simulink model "Hierarchical_Scheduler_2"  (Simulink 7.3)
settings: Solver=ode45  StartTime=0.0  StopTime=35000  RelTol=1e-3
model workspace: external: M-Code (data not in the file)
undefined symbols (not defined in the file or in its folder): D1, D2, D3, DiscIntNeverNeededParam, Sub, T1, T2, T3
libraries: simulink x3
settings Model: Creator=nmd01  LastModifiedBy=nmd01

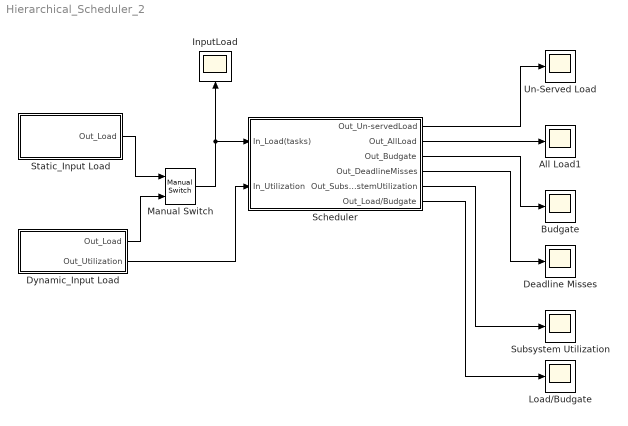
== system Hierarchical_Scheduler_2 ==
  All Load1 : Scope
      settings: SaveName=Utilization1  DataFormat=Array
  Budgate : Scope
      settings: SaveName=Utilization2  DataFormat=Array
  Deadline Misses : Scope
      settings: SaveName=Utilization11  DataFormat=Array
  Dynamic_Input Load : Subsystem
  InputLoad : Scope
      settings: SaveName=Utilization3  DataFormat=Array
  Load/Budgate : Scope
      settings: SaveName=Utilization13  DataFormat=Array
  Manual Switch : simulink/Signal Routing/Manual Switch  SystemSampleTime=-1  sw=1  action=0  varsize=off
  Scheduler : Subsystem
  Static_Input Load : Subsystem
  Subsystem Utilization : Scope
      settings: SaveName=Utilization12  DataFormat=Array
  Un-Served Load : Scope
      settings: SaveName=h  DataFormat=Array
  wires:
  Scheduler/1(Out_Un-servedLoad) -> Un-Served Load/1
  Scheduler/3(Out_Budgate) -> Budgate/1
  Static_Input Load/1(Out_Load) -> Manual Switch/1
  Dynamic_Input Load/1(Out_Load) -> Manual Switch/2
  Manual Switch/1 -> Scheduler/1(In_Load(tasks)), InputLoad/1
  Dynamic_Input Load/2(Out_Utilization) -> Scheduler/2(In_Utilization)
  Scheduler/4(Out_DeadlineMisses) -> Deadline Misses/1
  Scheduler/5(Out_SubsystemUtilization) -> Subsystem Utilization/1
  Scheduler/2(Out_AllLoad) -> All Load1/1
  Scheduler/6(Out_Load/Budgate) -> Load/Budgate/1

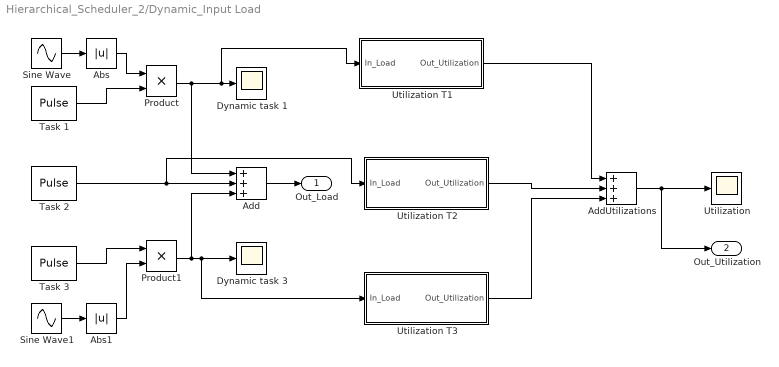
== system Hierarchical_Scheduler_2/Dynamic_Input Load ==
  Abs : Abs  OutDataType=fixdt(1, 16)  OutScaling=2^0
  Abs1 : Abs  OutDataType=fixdt(1, 16)  OutScaling=2^0
  Add : Sum  Inputs=+++  OutDataType=fixdt(1, 16)  OutScaling=2^-10
  AddUtilizations : Sum  Inputs=+++  OutDataType=fixdt(1, 16)  OutScaling=2^-10
  Dynamic task 1 : Scope
      settings: SaveName=Utilization6  DataFormat=Array
  Dynamic task 3 : Scope
      settings: SaveName=Utilization7  DataFormat=Array
  Product : Product  OutDataType=fixdt(1, 16)  OutScaling=2^0  SampleTime=1  RndMeth=Zero
  Product1 : Product  OutDataType=fixdt(1, 16)  OutScaling=2^0  SampleTime=1  RndMeth=Zero
  Sine Wave : Sin  Amplitude=1  Bias=0  Frequency=1  Phase=0  Samples=10  SampleTime=0  Offset=0
  Sine Wave1 : Sin  Amplitude=1  Bias=0  Frequency=3  Phase=0  Samples=10  SampleTime=0  Offset=0
  Task 1 : DiscretePulseGenerator  PulseType=Time based  Amplitude=5  Period=T1  PulseWidth=1  PhaseDelay=D1  SampleTime=1
  Task 2 : DiscretePulseGenerator  PulseType=Time based  Amplitude=2  Period=T2  PulseWidth=1  PhaseDelay=D2  SampleTime=1
  Task 3 : DiscretePulseGenerator  PulseType=Time based  Amplitude=1  Period=T3  PulseWidth=1  PhaseDelay=D3  SampleTime=1
  Utilization : Scope
      settings: SaveName=Utilization8  DataFormat=Array
  Utilization T1 : Subsystem
  Utilization T2 : Subsystem
  Utilization T3 : Subsystem
  Out_Load : Outport  OutDataType=fixdt(1, 16)  OutScaling=2^0
  Out_Utilization : Outport  Port=2  OutDataType=fixdt(1, 16)  OutScaling=2^0
  wires:
  Add/1 -> Out_Load/1
  Task 2/1 -> Add/2, Utilization T2/1(In_Load)
  Sine Wave/1 -> Abs/1
  Abs/1 -> Product/1
  Task 1/1 -> Product/2
  Product/1 -> Add/1, Dynamic task 1/1, Utilization T1/1(In_Load)
  Sine Wave1/1 -> Abs1/1
  Task 3/1 -> Product1/1
  Abs1/1 -> Product1/2
  Product1/1 -> Add/3, Dynamic task 3/1, Utilization T3/1(In_Load)
  Utilization T1/1(Out_Utilization) -> AddUtilizations/1
  Utilization T2/1(Out_Utilization) -> AddUtilizations/2
  Utilization T3/1(Out_Utilization) -> AddUtilizations/3
  AddUtilizations/1 -> Utilization/1, Out_Utilization/1

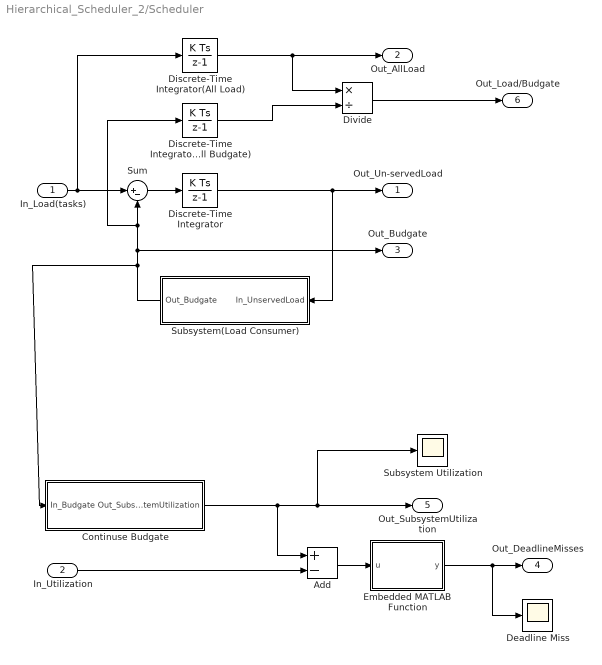
== system Hierarchical_Scheduler_2/Scheduler ==
  In_Load(tasks) : Inport  OutDataType=fixdt(1, 16)  OutScaling=2^0
  In_Utilization : Inport  Port=2  OutDataType=fixdt(1, 16)  OutScaling=2^0
  Add : Sum  Inputs=+-  OutDataType=fixdt(1, 16)  OutScaling=2^-10
  Continuse Budgate : Subsystem
  Deadline Miss : Scope
      settings: SaveName=Utilization10  DataFormat=Array
  Discrete-Time Integrator : DiscreteIntegrator  OutDataType=fixdt(1, 16)  OutScaling=2^0  LimitOutput=on  LowerSaturationLimit=0  ICPrevOutput=DiscIntNeverNeededParam  ICPrevScaledInput=DiscIntNeverNeededParam
  Discrete-Time Integrator(All Budgate) : DiscreteIntegrator  OutDataType=fixdt(1, 16)  OutScaling=2^0  LowerSaturationLimit=0  ICPrevOutput=DiscIntNeverNeededParam  ICPrevScaledInput=DiscIntNeverNeededParam
  Discrete-Time Integrator(All Load) : DiscreteIntegrator  OutDataType=fixdt(1, 16)  OutScaling=2^0  LowerSaturationLimit=0  ICPrevOutput=DiscIntNeverNeededParam  ICPrevScaledInput=DiscIntNeverNeededParam
  Divide : Product  Inputs=*/  OutDataType=fixdt(1, 16)  OutScaling=2^-10
  Embedded MATLAB Function : Stateflow chart
  Subsystem Utilization : Scope
      settings: SaveName=Utilization9  DataFormat=Array
  Subsystem(Load Consumer) : Subsystem
  Sum : Sum  Inputs=|+-  OutDataType=fixdt(1, 16)  OutScaling=2^0  SampleTime=1
  Out_Un-servedLoad : Outport  OutDataType=fixdt(1, 16)  OutScaling=2^0
  Out_AllLoad : Outport  Port=2  OutDataType=fixdt(1, 16)  OutScaling=2^0
  Out_Budgate : Outport  Port=3  OutDataType=fixdt(1, 16)  OutScaling=2^0
  Out_DeadlineMisses : Outport  Port=4  OutDataType=fixdt(1, 16)  OutScaling=2^0
  Out_SubsystemUtilization : Outport  Port=5  OutDataType=fixdt(1, 16)  OutScaling=2^0
  Out_Load/Budgate : Outport  Port=6  OutDataType=fixdt(1, 16)  OutScaling=2^0
  wires:
  In_Load(tasks)/1 -> Sum/1, Discrete-Time Integrator(All Load)/1
  Sum/1 -> Discrete-Time Integrator/1
  Discrete-Time Integrator/1 -> Out_Un-servedLoad/1, Subsystem(Load Consumer)/1(In_UnservedLoad)
  Subsystem(Load Consumer)/1(Out_Budgate) -> Out_Budgate/1, Sum/2, Discrete-Time Integrator(All Budgate)/1, Continuse Budgate/1(In_Budgate)
  Continuse Budgate/1(Out_SubsystemUtilization) -> Add/1, Subsystem Utilization/1, Out_SubsystemUtilization/1
  In_Utilization/1 -> Add/2
  Discrete-Time Integrator(All Load)/1 -> Out_AllLoad/1, Divide/1
  Divide/1 -> Out_Load/Budgate/1
  Discrete-Time Integrator(All Budgate)/1 -> Divide/2
  Add/1 -> Embedded MATLAB Function/1(u)
  Embedded MATLAB Function/1(y) -> Out_DeadlineMisses/1, Deadline Miss/1

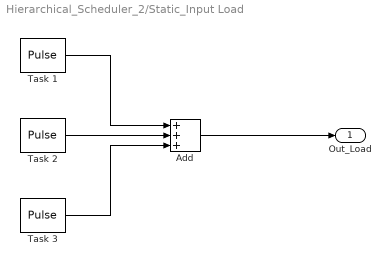
== system Hierarchical_Scheduler_2/Static_Input Load ==
  Add : Sum  Inputs=+++  OutDataType=fixdt(1, 16)  OutScaling=2^-10
  Task 1 : DiscretePulseGenerator  PulseType=Time based  Amplitude=3  Period=T1  PulseWidth=1  PhaseDelay=D1  SampleTime=1
  Task 2 : DiscretePulseGenerator  PulseType=Time based  Amplitude=2  Period=T2  PulseWidth=1  PhaseDelay=D2  SampleTime=1
  Task 3 : DiscretePulseGenerator  PulseType=Time based  Amplitude=1  Period=T3  PulseWidth=D3  PhaseDelay=0  SampleTime=1
  Out_Load : Outport  OutDataType=fixdt(1, 16)  OutScaling=2^0
  wires:
  Add/1 -> Out_Load/1
  Task 1/1 -> Add/1
  Task 2/1 -> Add/2
  Task 3/1 -> Add/3

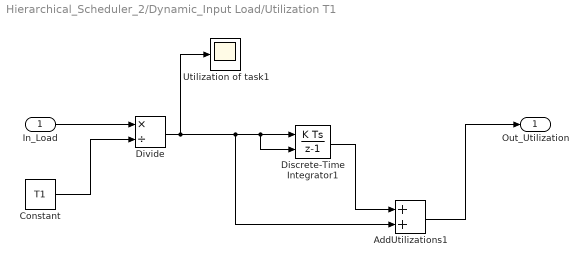
== system Hierarchical_Scheduler_2/Dynamic_Input Load/Utilization T1 ==
  In_Load : Inport  OutDataType=fixdt(1, 16)  OutScaling=2^0
  AddUtilizations1 : Sum  OutDataType=fixdt(1, 16)  OutScaling=2^-10
  Constant : Constant  Value=T1  OutDataType=fixdt(1, 16)  OutScaling=2^0
  Discrete-Time Integrator1 : DiscreteIntegrator  ExternalReset=rising  OutDataType=fixdt(1, 16)  OutScaling=2^0  ICPrevOutput=DiscIntNeverNeededParam  ICPrevScaledInput=DiscIntNeverNeededParam
  Divide : Product  Inputs=*/  OutDataType=fixdt(1, 16)  OutScaling=2^-10
  Utilization of task1 : Scope
      settings: SaveName=Utilization  DataFormat=Array
  Out_Utilization : Outport  OutDataType=fixdt(1, 16)  OutScaling=2^0
  wires:
  In_Load/1 -> Divide/1
  Constant/1 -> Divide/2
  Divide/1 -> Discrete-Time Integrator1/1, Discrete-Time Integrator1/2, AddUtilizations1/2, Utilization of task1/1
  Discrete-Time Integrator1/1 -> AddUtilizations1/1
  AddUtilizations1/1 -> Out_Utilization/1

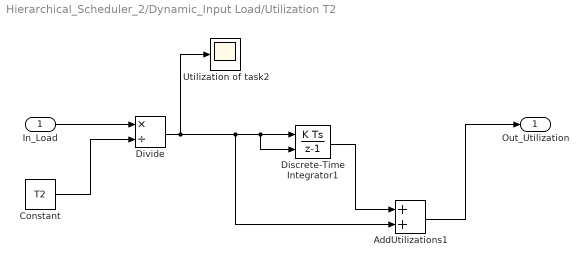
== system Hierarchical_Scheduler_2/Dynamic_Input Load/Utilization T2 ==
  In_Load : Inport  OutDataType=fixdt(1, 16)  OutScaling=2^0
  AddUtilizations1 : Sum  OutDataType=fixdt(1, 16)  OutScaling=2^-10
  Constant : Constant  Value=T2  OutDataType=fixdt(1, 16)  OutScaling=2^0
  Discrete-Time Integrator1 : DiscreteIntegrator  ExternalReset=rising  OutDataType=fixdt(1, 16)  OutScaling=2^0  ICPrevOutput=DiscIntNeverNeededParam  ICPrevScaledInput=DiscIntNeverNeededParam
  Divide : Product  Inputs=*/  OutDataType=fixdt(1, 16)  OutScaling=2^-10
  Utilization of task2 : Scope
      settings: SaveName=Utilization  DataFormat=Array
  Out_Utilization : Outport  OutDataType=fixdt(1, 16)  OutScaling=2^0
  wires:
  AddUtilizations1/1 -> Out_Utilization/1
  Discrete-Time Integrator1/1 -> AddUtilizations1/1
  Divide/1 -> Utilization of task2/1, AddUtilizations1/2, Discrete-Time Integrator1/2, Discrete-Time Integrator1/1
  Constant/1 -> Divide/2
  In_Load/1 -> Divide/1

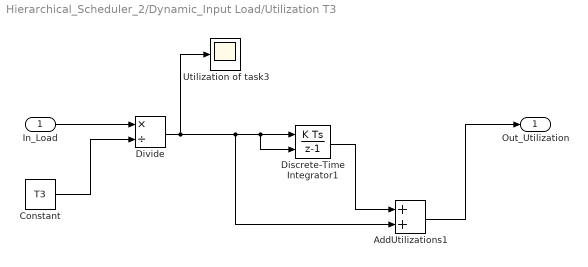
== system Hierarchical_Scheduler_2/Dynamic_Input Load/Utilization T3 ==
  In_Load : Inport  OutDataType=fixdt(1, 16)  OutScaling=2^0
  AddUtilizations1 : Sum  OutDataType=fixdt(1, 16)  OutScaling=2^-10
  Constant : Constant  Value=T3  OutDataType=fixdt(1, 16)  OutScaling=2^0
  Discrete-Time Integrator1 : DiscreteIntegrator  ExternalReset=rising  OutDataType=fixdt(1, 16)  OutScaling=2^0  ICPrevOutput=DiscIntNeverNeededParam  ICPrevScaledInput=DiscIntNeverNeededParam
  Divide : Product  Inputs=*/  OutDataType=fixdt(1, 16)  OutScaling=2^-10
  Utilization of task3 : Scope
      settings: SaveName=Utilization  DataFormat=Array
  Out_Utilization : Outport  OutDataType=fixdt(1, 16)  OutScaling=2^0
  wires:
  In_Load/1 -> Divide/1
  Constant/1 -> Divide/2
  Divide/1 -> Discrete-Time Integrator1/1, Discrete-Time Integrator1/2, AddUtilizations1/2, Utilization of task3/1
  Discrete-Time Integrator1/1 -> AddUtilizations1/1
  AddUtilizations1/1 -> Out_Utilization/1

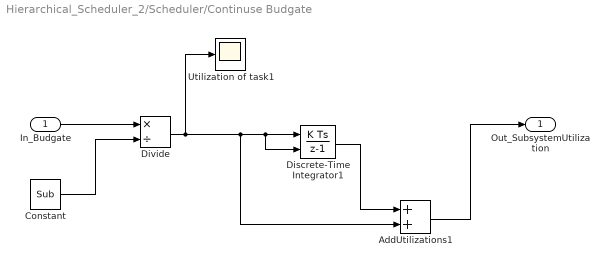
== system Hierarchical_Scheduler_2/Scheduler/Continuse Budgate ==
  In_Budgate : Inport  OutDataType=fixdt(1, 16)  OutScaling=2^0
  AddUtilizations1 : Sum  OutDataType=fixdt(1, 16)  OutScaling=2^-10
  Constant : Constant  Value=Sub  OutDataType=fixdt(1, 16)  OutScaling=2^0
  Discrete-Time Integrator1 : DiscreteIntegrator  ExternalReset=rising  OutDataType=fixdt(1, 16)  OutScaling=2^0  ICPrevOutput=DiscIntNeverNeededParam  ICPrevScaledInput=DiscIntNeverNeededParam
  Divide : Product  Inputs=*/  OutDataType=fixdt(1, 16)  OutScaling=2^-10
  Utilization of task1 : Scope
      settings: SaveName=Utilization  DataFormat=Array
  Out_SubsystemUtilization : Outport  OutDataType=fixdt(1, 16)  OutScaling=2^0
  wires:
  In_Budgate/1 -> Divide/1
  Discrete-Time Integrator1/1 -> AddUtilizations1/1
  AddUtilizations1/1 -> Out_SubsystemUtilization/1
  Divide/1 -> Discrete-Time Integrator1/1, Discrete-Time Integrator1/2, AddUtilizations1/2, Utilization of task1/1
  Constant/1 -> Divide/2

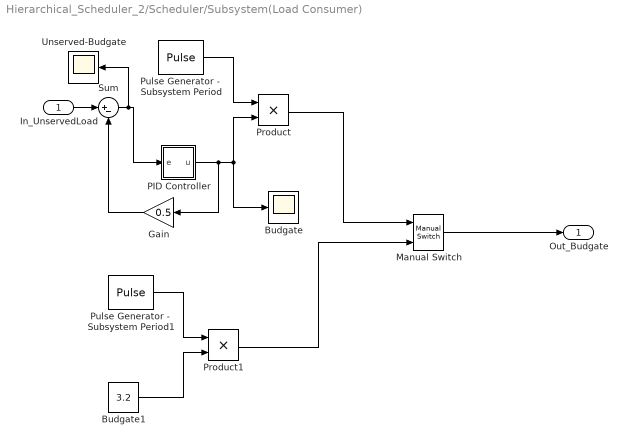
== system Hierarchical_Scheduler_2/Scheduler/Subsystem(Load Consumer) ==
  In_UnservedLoad : Inport  OutDataType=fixdt(1, 16)  OutScaling=2^0
  Budgate : Scope
      settings: SaveName=Utilization4  DataFormat=Array
  Budgate1 : Constant  Value=3.2  OutDataType=fixdt(1, 16)  OutScaling=2^0
  Gain : Gain  Gain=0.5  ParameterDataType=fixdt(1, 16)  ParameterScaling=2^0  OutDataType=fixdt(1, 16)  OutScaling=2^0
  Manual Switch : simulink/Signal Routing/Manual Switch  SystemSampleTime=-1  sw=1  action=0  varsize=off
  PID Controller : Subsystem  AncestorBlock=simulink_extras/Additional Linear/PID Controller  mask(PID Controller){P=.01, I=.001, D=0}
      mask prompts: P "Proportional:"; I "Integral:"; D "Derivative:"
      mask help:
      | Enter expressions for proportional, integral, and derivative terms.
      | P+I/s+Ds
      mask Help: This block implements a PID controller where parameters are entered for the Proportional, Integral and Derivative terms. Unmask this block to see how it works. The derivative term is implemented using a true derivative block.
      mask Display: disp('PID')
  Product : Product  OutDataType=fixdt(1, 16)  OutScaling=2^0  SampleTime=1  RndMeth=Zero
  Product1 : Product  OutDataType=fixdt(1, 16)  OutScaling=2^0  SampleTime=1  RndMeth=Zero
  Pulse Generator -  Subsystem Period : DiscretePulseGenerator  PulseType=Time based  Amplitude=1  Period=Sub  PulseWidth=1  PhaseDelay=0  SampleTime=1
  Pulse Generator -  Subsystem Period1 : DiscretePulseGenerator  PulseType=Time based  Amplitude=1  Period=Sub  PulseWidth=1  PhaseDelay=0  SampleTime=1
  Sum : Sum  Inputs=|+-  OutDataType=fixdt(1, 16)  OutScaling=2^0  SampleTime=1
  Unserved-Budgate : Scope
      settings: SaveName=Utilization5  DataFormat=Array
  Out_Budgate : Outport  OutDataType=fixdt(1, 16)  OutScaling=2^0
  wires:
  Pulse Generator -  Subsystem Period/1 -> Product/1
  PID Controller/1(u) -> Product/2, Budgate/1, Gain/1
  In_UnservedLoad/1 -> Sum/1
  Sum/1 -> PID Controller/1(e), Unserved-Budgate/1
  Pulse Generator -  Subsystem Period1/1 -> Product1/1
  Budgate1/1 -> Product1/2
  Product/1 -> Manual Switch/1
  Product1/1 -> Manual Switch/2
  Manual Switch/1 -> Out_Budgate/1
  Gain/1 -> Sum/2

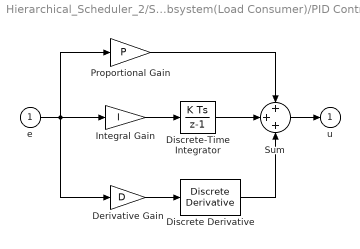
== system Hierarchical_Scheduler_2/Scheduler/Subsystem(Load Consumer)/PID Controller ==
  e : Inport  OutDataType=sfix(16)  OutScaling=2^0
  Derivative Gain : Gain  Gain=D  ParameterDataType=sfix(16)  ParameterScaling=2^0  OutDataType=sfix(16)  OutScaling=2^0  SampleTime=Sub  SaturateOnIntegerOverflow=on  OutDataTypeStr=Inherit: Same as input  ParamDataTypeStr=Inherit: Same as input
  Discrete Derivative : simulink/Discrete/Discrete Derivative  SystemSampleTime=-1  gainval=1.0  ICPrevScaledInput=0.0  OutMin=[]  OutMax=[]  OutDataType=fixdt(1, 16)  OutScaling=2^-10  DoSatur=off
  Discrete-Time Integrator : DiscreteIntegrator  InitialCondition=1  SampleTime=Sub  OutDataType=fixdt(1, 16)  OutScaling=2^0  ICPrevOutput=DiscIntNeverNeededParam  ICPrevScaledInput=DiscIntNeverNeededParam
  Integral Gain : Gain  Gain=I  ParameterDataType=sfix(16)  ParameterScaling=2^0  OutDataType=sfix(16)  OutScaling=2^0  SampleTime=Sub  SaturateOnIntegerOverflow=on  OutDataTypeStr=Inherit: Same as input  ParamDataTypeStr=Inherit: Same as input
  Proportional Gain : Gain  Gain=P  ParameterDataType=sfix(16)  ParameterScaling=2^0  OutDataType=sfix(16)  OutScaling=2^0  SampleTime=Sub  SaturateOnIntegerOverflow=on  OutDataTypeStr=Inherit: Same as input  ParamDataTypeStr=Inherit: Same as input
  Sum : Sum  Inputs=+++  OutDataType=sfix(16)  OutScaling=2^0  SaturateOnIntegerOverflow=on  InputSameDT=on  OutDataTypeStr=Inherit: Same as first input
  u : Outport  OutDataType=sfix(16)  OutScaling=2^0  InitialOutput=0
  wires:
  Integral Gain/1 -> Discrete-Time Integrator/1
  Proportional Gain/1 -> Sum/1
  Discrete-Time Integrator/1 -> Sum/2
  Discrete Derivative/1 -> Sum/3
  e/1 -> Derivative Gain/1, Proportional Gain/1, Integral Gain/1
  Sum/1 -> u/1
  Derivative Gain/1 -> Discrete Derivative/1

== matlab function Scheduler/Embedded MATLAB Function ==
  data: u input double; y output double
function y = fcn(u)
%#eml
if u<0
    y=-u;
else
y = 0;
end
